simulink model "Motor_Position_Modelw_friction_6_open_loop"  (R2013b)
settings: Solver=ode45  StartTime=0.0  StopTime=16  FixedStep=.0001  RelTol=1e-6  AbsTol=1e-6
values from neighbouring files (symbols this model uses):
  Fo = 1    [Motor_Position_Modelw_friction_6m_Lab.m]
  Gain = 23    [Motor_Position_Modelw_friction_6m_Lab.m]
  Input_Amplitude = .1    (= 0.1)    [Motor_Position_Modelw_friction_6m_Lab.m]
  Input_Frequency = 2*pi/Period    (= 6.28318530718)    [Motor_Position_Modelw_friction_6m_Lab.m]
  Kinetic_friction_Force = 1000    [Motor_Position_Modelw_friction_6m_Lab.m]
  Kinetic_friction_transition_rate = 1000    [Motor_Position_Modelw_friction_6m_Lab.m]
  Omegan = 2*pi*frequency_n    (= 50)    [Motor_Position_Modelw_friction_6m_Lab.m]
  Zeta = 0.74    [Motor_Position_Modelw_friction_6m_Lab.m]
settings Model: Creator=davet  LastModifiedBy=davet
settings DataIOCC: SignalLoggingSaveFormat=ModelDataLogs  SignalLoggingName=sigsOut
settings OptimizationCC: BlockReduction=off  BooleanDataType=off  ExpressionDepthLimit=2147483647
settings DebuggingCC: SaveWithParameterizedLinksMsg=none  SignalResolutionControl=TryResolveAllWithWarning  SolverPrmCheckMsg=none  MultiTaskDSMMsg=warning  MultiTaskCondExecSysMsg=none  FcnCallInpInsideContextMsg=UseLocalSettings  StateNameClashWarn=warning
settings HardwareCC: TargetUnknown=on
settings RTWCC: IncludeERTFirstTime=on
settings GRTTargetCC: ModelReferenceCompliant=off  ParMdlRefBuildCompliant=off  CompOptLevelCompliant=off  ConcurrentExecutionCompliant=off  CombineOutputUpdateFcns=off  MatFileLogging=off  GRTInterface=on

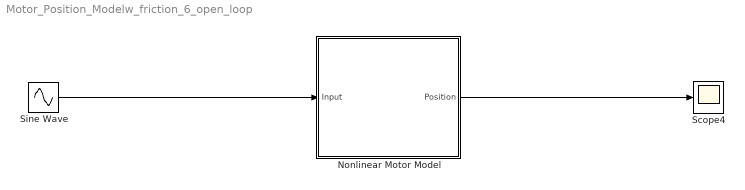
== system Motor_Position_Modelw_friction_6_open_loop ==
  Nonlinear Motor Model : Subsystem
  Scope4 : Scope
      settings: SaveName=ScopeData4
  Sine Wave : Sin  Amplitude=Input_Amplitude  Frequency=Input_Frequency  SampleTime=0
  wires:
  Nonlinear Motor Model/1(Position) -> Scope4/1
  Sine Wave/1 -> Nonlinear Motor Model/1(Input)

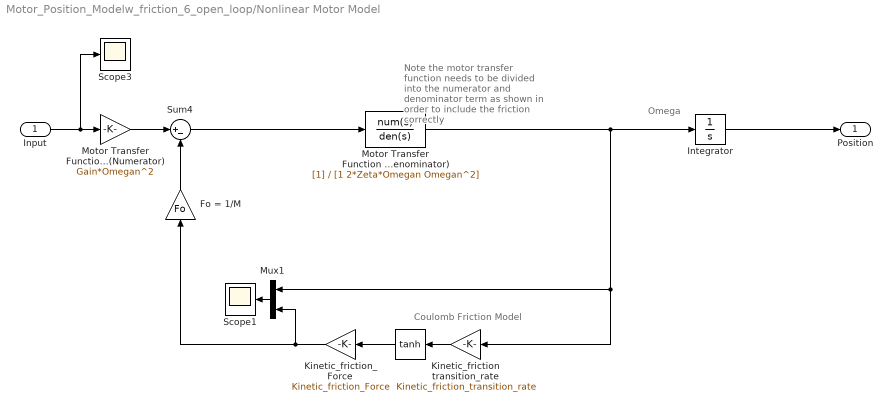
== system Motor_Position_Modelw_friction_6_open_loop/Nonlinear Motor Model ==
  note: Omega
  note: Coulomb Friction Model
  note: Note the motor transfer function needs to be divided
      |  into the numerator and denominator term as shown
      | in order to include the friction correctly
  Input : Inport
  " " : Trigonometry  Operator=tanh
  Fo = 1/M : Gain  Gain=Fo  SaturateOnIntegerOverflow=on  OutDataTypeStr=Inherit: Same as input  ParamDataTypeStr=Inherit: Same as input
  Integrator : Integrator
  Kinetic_friction transition_rate : Gain  Gain=Kinetic_friction_transition_rate
  Kinetic_friction_Force : Gain  Gain=Kinetic_friction_Force
  Motor Transfer Function (Numerator) : Gain  Gain=Gain*Omegan^2  SaturateOnIntegerOverflow=on  OutDataTypeStr=Inherit: Same as input  ParamDataTypeStr=Inherit: Same as input
  Motor Transfer Function (Denominator) : TransferFcn  Denominator=[1 2*Zeta*Omegan Omegan^2]
  Mux1 : Mux  Inputs=2
  Scope1 : Scope
      settings: TimeRange=20  YMin=-0.2  YMax=0.2
  Scope3 : Scope
      settings: TimeRange=20  YMin=-0.2  YMax=0.2  SaveName=ScopeData3
  Sum4 : Sum  Inputs=|+-  SaturateOnIntegerOverflow=on  InputSameDT=on  OutDataTypeStr=Inherit: Same as first input
  Position : Outport
  wires:
  Motor Transfer Function (Denominator)/1 -> Integrator/1, Kinetic_friction transition_rate/1, Mux1/1
  Input/1 -> Scope3/1, Motor Transfer Function (Numerator)/1
  " "/1 -> Kinetic_friction_Force/1
  Kinetic_friction transition_rate/1 -> " "/1
  Kinetic_friction_Force/1 -> Mux1/2, Fo = 1/M/1
  Mux1/1 -> Scope1/1
  Fo = 1/M/1 -> Sum4/2
  Sum4/1 -> Motor Transfer Function (Denominator)/1
  Motor Transfer Function (Numerator)/1 -> Sum4/1
  Integrator/1 -> Position/1
